simulink model "Antecipativo"  (R2018a)
settings: Solver=VariableStepAuto  StartTime=0.0  StopTime=10000  RelTol=1e-3
values from neighbouring files (symbols this model uses):
  K = 0.36783    [carregaDados.m]    (also in carregaDadosDoModelo.m = 0.01332; carregaDadosSimulacao.m = 0.01)
  Ki = 13 * Kp    (= 1.56)    [carregaDados.m]    (also in carregaDadosSimulacao.m)
  Kp = 0.12    [carregaDados.m]    (also in carregaDadosSimulacao.m)
  tau = 13.314    [carregaDados.m]    (also in carregaDadosSimulacao.m)
  td = 0.065    [carregaDados.m]    (also in carregaDadosSimulacao.m = 5)
libraries: simulink x1
settings Model: Creator=alexa  LastModifiedBy=alexa

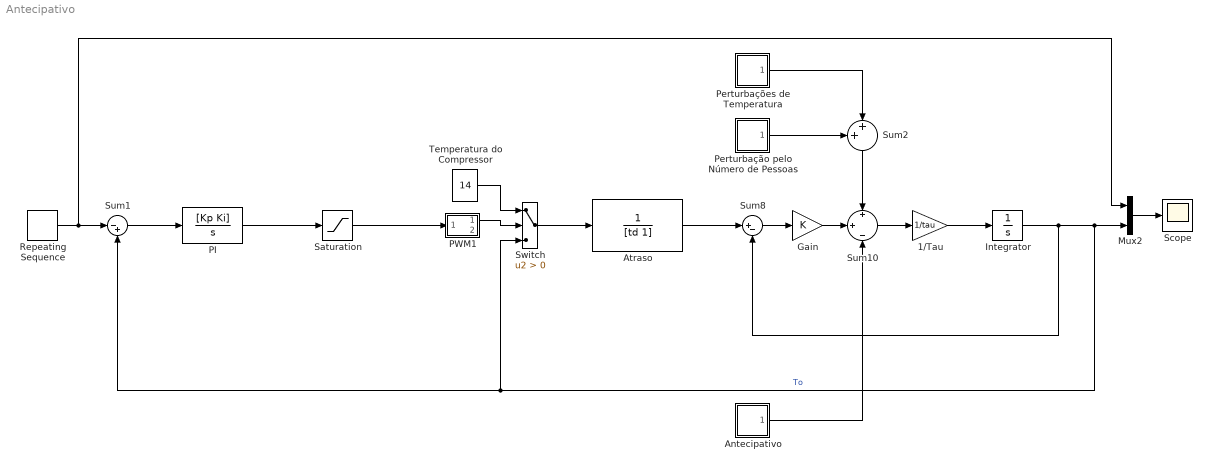
== system Antecipativo ==
  "1/Tau " : Gain  Gain=1/tau
  Antecipativo : Subsystem
  Atraso : TransferFcn  Denominator=[td 1]
  Gain : Gain  Gain=K
  Integrator : Integrator  InitialCondition=24
  Mux2 : Mux  Inputs=2
  PI : TransferFcn  Numerator=[Kp Ki]  Denominator=[1 0]
  PWM1 : Subsystem  mask(Pulse Generator){period=600, amplitude=1, start=0}
      mask prompts: period "Period (secs):"; start "Start time:"
      mask help: Pulse Generator
      mask Help: Pulse generator which ensures pulse transitions are hit. Provides a vector of pulses when the height is entered as a vector.  Unmask to see how it works.
      mask Display: plot(0,0,100,100,[95,90,90,75,75,60,60,45,45,30,30,15,15,5],[25,25,75,75,25,25,75,75,25,25,75,75,25,25]);
  Perturbação pelo Número de Pessoas : Subsystem
  Perturbações de Temperatura : Subsystem
  Repeating Sequence : simulink/Sources/Repeating Sequence  rep_seq_t=[0 200 201 10000]  rep_seq_y=[30 30 22 22]
  Saturation : Saturate  UpperLimit=1  LowerLimit=-1
  Scope : Scope
  Sum1 : Sum  Inputs=|-+
  Sum10 : Sum  Inputs=+|+|-
  Sum2 : Sum  Inputs=++|
  Sum8 : Sum  Inputs=|+-
  Switch : Switch  Criteria=u2 > Threshold
  Temperatura do Compressor : Constant  Value=14
  wires:
  PWM1/1(Out1) -> Switch/2
  Temperatura do Compressor/1 -> Switch/1
  Integrator/1 -> Sum8/2, Mux2/2, Switch/3, Sum1/2  "To"
  Sum8/1 -> Gain/1
  Repeating Sequence/1 -> Sum1/1, Mux2/1
  Switch/1 -> Atraso/1
  "1/Tau "/1 -> Integrator/1
  Mux2/1 -> Scope/1
  Sum1/1 -> PI/1
  Saturation/1 -> PWM1/1(In1)
  Atraso/1 -> Sum8/1
  Sum10/1 -> "1/Tau "/1
  PI/1 -> Saturation/1
  Perturbações de Temperatura/1(Out1) -> Sum2/2
  Perturbação pelo Número de Pessoas/1(Out1) -> Sum2/1
  Gain/1 -> Sum10/2
  Antecipativo/1(Out1) -> Sum10/3
  Sum2/1 -> Sum10/1

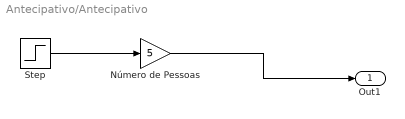
== system Antecipativo/Antecipativo ==
  Número de Pessoas : Gain  Gain=5
  Step : Step  Time=0  After=0.2  SampleTime=0
  Out1 : Outport
  wires:
  Step/1 -> Número de Pessoas/1
  Número de Pessoas/1 -> Out1/1

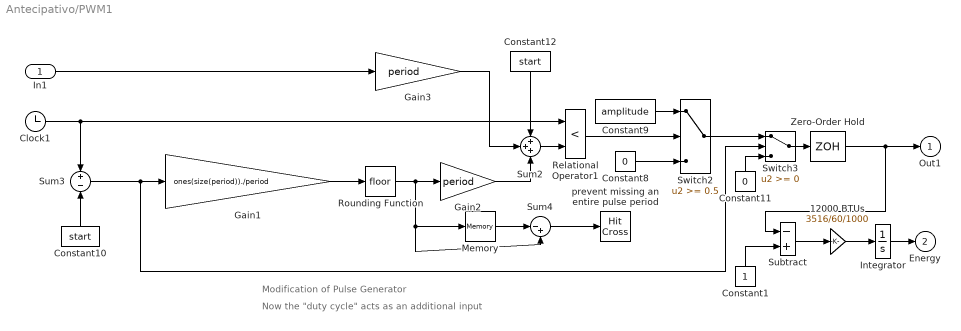
== system Antecipativo/PWM1 ==
  note: Now the "duty cycle" acts as an additional input
  note: Modification of Pulse Generator
  In1 : Inport
  12000 BTUs : Gain  Gain=3516/60/1000
  Clock1 : Clock
  Constant1 : Constant
  Constant10 : Constant  Value=start
  Constant11 : Constant  Value=0
  Constant12 : Constant  Value=start
  Constant8 : Constant  Value=0
  Constant9 : Constant  Value=amplitude
  Gain1 : Gain  Gain=ones(size(period))./period  SaturateOnIntegerOverflow=on  OutDataTypeStr=Inherit: Same as input  ParamDataTypeStr=Inherit: Same as input
  Gain2 : Gain  Gain=period  SaturateOnIntegerOverflow=on  OutDataTypeStr=Inherit: Same as input  ParamDataTypeStr=Inherit: Same as input
  Gain3 : Gain  Gain=period  SaturateOnIntegerOverflow=on  OutDataTypeStr=Inherit: Same as input  ParamDataTypeStr=Inherit: Same as input
  Integrator : Integrator
  Memory : Memory
  Relational Operator1 : RelationalOperator  Operator=<  RndMeth=Nearest  InputSameDT=on
  Rounding Function : Rounding
  Subtract : Sum  Inputs=-+
  Sum2 : Sum  Inputs=+++  SaturateOnIntegerOverflow=on  InputSameDT=on  OutDataTypeStr=Inherit: Same as first input
  Sum3 : Sum  Inputs=+-  SaturateOnIntegerOverflow=on  InputSameDT=on  OutDataTypeStr=Inherit: Same as first input
  Sum4 : Sum  Inputs=|-+  SaturateOnIntegerOverflow=on  InputSameDT=on  OutDataTypeStr=Inherit: Same as first input
  Switch2 : Switch  Threshold=0.5  SaturateOnIntegerOverflow=on  InputSameDT=on
  Switch3 : Switch  SaturateOnIntegerOverflow=on  InputSameDT=on
  Zero-Order Hold : ZeroOrderHold  SampleTime=.1
  prevent missing an entire pulse period : HitCross  HitCrossingOffset=1  ShowOutputPort=off
  Out1 : Outport
  Energy : Outport  Port=2
  wires:
  Gain3/1 -> Sum2/2
  Constant12/1 -> Sum2/1
  In1/1 -> Gain3/1
  Gain2/1 -> Sum2/3
  Constant10/1 -> Sum3/2
  Sum3/1 -> Gain1/1, Switch3/2
  Clock1/1 -> Relational Operator1/1, Sum3/1
  Sum2/1 -> Relational Operator1/2
  Gain1/1 -> Rounding Function/1
  Rounding Function/1 -> Sum4/2, Memory/1, Gain2/1
  Switch3/1 -> Zero-Order Hold/1
  Relational Operator1/1 -> Switch2/2
  Constant8/1 -> Switch2/3
  Constant9/1 -> Switch2/1
  Constant11/1 -> Switch3/3
  Switch2/1 -> Switch3/1
  Sum4/1 -> prevent missing an entire pulse period/1
  Memory/1 -> Sum4/1
  Zero-Order Hold/1 -> Out1/1, Subtract/1
  Integrator/1 -> Energy/1
  Constant1/1 -> Subtract/2
  12000 BTUs/1 -> Integrator/1
  Subtract/1 -> 12000 BTUs/1

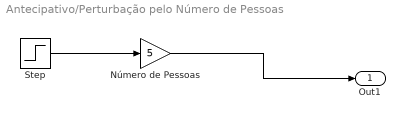
== system Antecipativo/Perturbação pelo Número de Pessoas ==
  Número de Pessoas : Gain  Gain=5
  Step : Step  Time=0  After=0.2  SampleTime=0
  Out1 : Outport
  wires:
  Step/1 -> Número de Pessoas/1
  Número de Pessoas/1 -> Out1/1

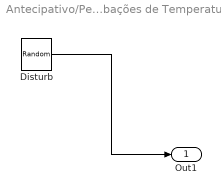
== system Antecipativo/Perturbações de Temperatura ==
  Disturb : UniformRandomNumber  Minimum=-0.25  Maximum=5  SampleTime=1
  Out1 : Outport
  wires:
  Disturb/1 -> Out1/1
